simulink model "blank_model_gcm48"  (R2021a)
settings: Solver=FixedStepDiscrete  StartTime=0.0  StopTime=10.0  FixedStep=0.005  RelTol=1e-3  EnableMultiTasking=on
PreLoadFcn:
  | try, model_open; catch, disp('Error occurred while executing model pre-load callback: model_open.m'); disp('Please assure that the MATLAB working directory is set to the model directory before opening.'); end
InitFcn:
  | try, model_open; catch, end
undefined symbols (not defined in the file): dataName, enumName, enumValue, GCM, raptor_get_safe_string, raptor_xcp_function
libraries: Raptor_lib x50, simulink x8
(part 1 of 2)
CloseFcn:
  | try, model_close; catch, end
settings Model: Raptor_Target=GCM-5605B-048-2104  Raptor_Calloc=NonVolatile (EEPROM)  RaptorUIDSize=4  RaptorBuildNum=3  Raptor_ecuaddr=11  Raptor_IsLiteMode=1  Creator=Ben  LastModifiedBy=siddh
settings SolverCC: AlgebraicLoopSolver=TrustRegion
settings DataIOCC: LimitDataPoints=on  SaveFormat=Array  SignalLoggingSaveFormat=ModelDataLogs  ReturnWorkspaceOutputs=off
settings OptimizationCC: DefaultParameterBehavior=Inlined  ExpressionDepthLimit=2147483647  InitFltsAndDblsToZero=on  LifeSpan=1  EfficientTunableParamExpr=on
settings DebuggingCC: SolverPrmCheckMsg=warning  InheritedTsInSrcMsg=none  FcnCallInpInsideContextMsg=warning  StateNameClashWarn=warning  SFUnexpectedBacktrackingDiag=warning  SFNoUnconditionalDefaultTransitionDiag=warning  SFExecutionAtInitializationDiag=none  SFMachineParentedDataDiag=warning  ArithmeticOperatorsInVariantConditions=warning
settings HardwareCC: ProdBitPerPointer=32  ProdBitPerSizeT=32  ProdBitPerPtrDiffT=32  ProdLargestAtomicInteger=Long  ProdLargestAtomicFloat=Double  ProdEndianess=BigEndian  ProdWordSize=32  ProdHWDeviceType=Freescale->MPC55xx  TargetIntDivRoundTo=Zero  TargetEndianess=BigEndian  ProdEqTarget=off
settings ModelReferenceCC: PropagateSignalLabelsOutOfModel=off
settings SFSimCC: SimUseLocalCustomCode=off  MATLABDynamicMemAlloc=off  CustomCodeUndefinedFunction=UseInterfaceOnly
settings RTWCC: Description=Raptor (tm)  SystemTargetFile=raptor.tlc  GenCodeOnly=on  MakeCommand=raptor_make_rtw  TemplateMakefile=raptor.tmf  RTWUseLocalCustomCode=off
settings CodeAppCC: IgnoreCustomStorageClasses=off  MaxIdLength=100  CustomSymbolStrType=$N$R$M  StateflowObjectComments=on  InternalIdentifier=Classic
settings STFCustomTargetCC: GenerateSampleERTMain=on  ModelReferenceCompliant=off  CombineOutputUpdateFcns=on  ERTCustomFileBanners=on  SupportContinuousTime=off  SupportNonInlinedSFcns=off  RemoveResetFunc=on  MATLABClassNameForMDSCustomization=Simulink.SoftwareTarget.ERTCustomization  GRTInterface=off  UseToolchainInfoCompliant=off  SystemTargetFile=raptor.tlc
settings ERTTargetCC: MultiwordLength=2048  GenerateSampleERTMain=on  ModelReferenceCompliant=off  ParMdlRefBuildCompliant=off  CompOptLevelCompliant=off  ConcurrentExecutionCompliant=off  ModelStepFunctionPrototypeControlCompliant=off  CPPClassGenCompliant=off  UseToolchainInfoCompliant=off  ExtModeMexFile=noextcomm  InlinedParameterPlacement=NonHierarchical  ERTCustomFileTemplate=example_file_process.tlc  ConvertIfToSwitch=off  SuppressUnreachableDefaultCases=off
settings ConfigComp: CovMetricSettings=dw  CovSaveCumulativeToWorkspaceVar=on  CovSaveSingleToWorkspaceVar=on  CovExternalEMLEnable=off  CovSFcnEnable=off

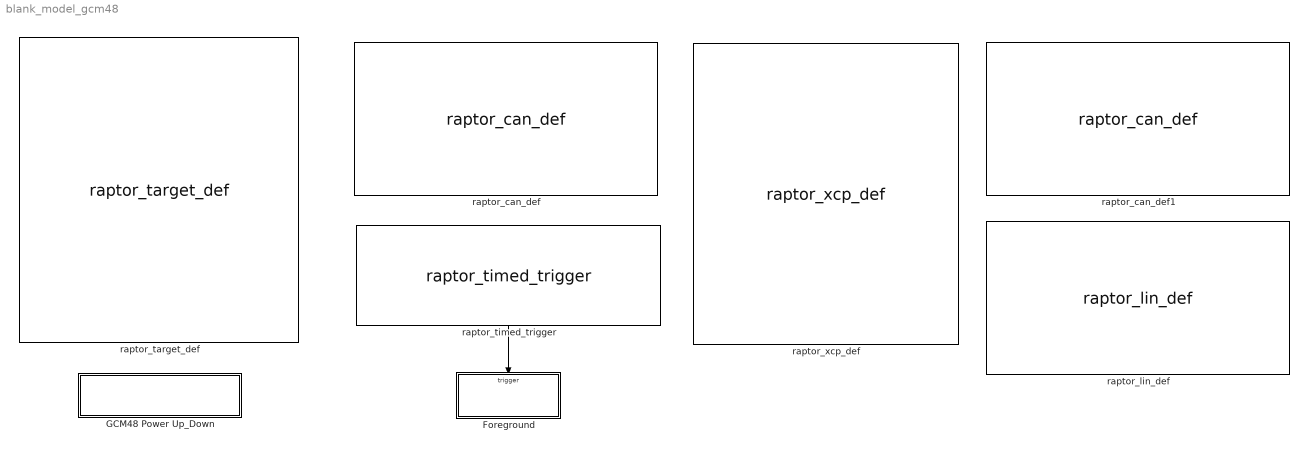
== system blank_model_gcm48 ==
  Foreground : Subsystem  TreatAsAtomicUnit=on
      mask init:
      | handles = get_param(gcb,'PortHandles');
      | portConnectivity = get_param(gcb,'PortConnectivity');
      | for i = 1:length(portConnectivity)
      |     if strcmp(portConnectivity(i).Type,'trigger')
      |         triggerBlk = portConnectivity(i).SrcBlock;
      |         triggerString = get_param(triggerBlk,'trigger');
      |         break;
      |     end
      | end
      | 
      | trigConfBlks = find_system(bdroot,'MaskType','Timed Trigger Configuration Block');
      | trigConfigFound = false;
      | for i = 1:length(trigConfBlks)
      |     if ~isempty(strfind(triggerString,raptor_get_param_eval(trigConfBlks{i},'trigger')))
      |         %if this if statement is met, it means, for example, the text
      |         %"Background" was found in the trigger name of "Backgroundx5"
      |         period_ms = raptor_get_param_eval(trigConfBlks{i},'period');
      |         trigConfigFound = true;
      |         break;
      |     end      
      | end
      | 
      | if ~trigConfigFound %no config defined
      |     switch triggerString
      |         case 'Second'
      |             period_ms = 1000;
      |         case 'Minute'
      |             period_ms = 60*1000;
      |         case 'Foreground'
      |             period_ms = 10;
      |         case 'Background'
      |             period_ms = 100;
      |     end
      | end    
      | 
      | switch triggerString(end-1:end)
      |     case 'x2' %Fgnd or Bgnd slowed by a factor of 2
      |         mult = 2;
      |     case 'x5'
      |         mult = 5;
      |     case '10'
      |         mult = 10;
      |     case '20'
      |         mult = 20;
      |     otherwise
      |         mult = 1;
      | end
      | samptime = period_ms/1000*mult;
      settings: RTWSystemCode=Nonreusable function
      mask Display: disp(['Sample Time:\n' num2str(samptime)])
  GCM48 Power Up_Down : Subsystem  mask{group='Diagnostics | Power Up_Down'}
  raptor_can_def : Raptor_lib/CAN/raptor_can_def  canBus='CAN1'  resourceValues=CAN1|CAN2|CAN3|CAN4|CAN5|CAN6|(None)  resource=CAN1  baudRateValues=33k|50k|100k|125k|200k|250k|333k|500k|667k|800k|1000k  baudRate=500k  enable_baud_rate_config=0  sim_func_name='ConfigureCANBaudRate'  createButton=[]  txQueueSize=20  rxQueueSize=16
      settings: SourceProductName=Raptor
  raptor_can_def1 : Raptor_lib/CAN/raptor_can_def  canBus='CAN2'  resourceValues=CAN1|CAN2|CAN3|CAN4|CAN5|CAN6|(None)  resource=CAN2  baudRateValues=125k|250k|500k|1000k  baudRate=500k  enable_baud_rate_config=0  sim_func_name='ConfigureCANBaudRate'  createButton=[]  txQueueSize=20  rxQueueSize=16
      settings: SourceProductName=Raptor
  raptor_lin_def : Raptor_lib/LIN/raptor_lin_def  linBus='LIN2'  resourceValues=LIN1|LIN2|LIN3|(None)  resource=LIN2  baudRateValues=1200|2400|4800|9600|10000|10400|19200  baudRate=10400  ldfFile='lin_example.ldf'  master=''  chooseLdf=[]
      settings: SourceProductName=Raptor
  raptor_target_def : Raptor_lib/Configuration/raptor_target_def  targetValues=BCM-5646-48-1404|DISP-VC128-1901|DISP-VC320L-1402|DISP-VC320-1204|DISP-VC800-1402|DISP-VC500-1904|DISP-VC700-2003|DISP-VC300R-2004|GCM-5634M-070-1459|GCM-5634M-070-1559|GCM-5634M-070-1562|ECM-1793-196-1503|GCM-1793-196-1503|GCM-5605B-048-1906|GCM-5605B-048-2104|GCM-5607B-80-1901|GCM-5607B-80-1903|GCM-5607B-80-2001|RCM-5743R-080-2005|RCM-5743R-080-2106|UAS-5743R-047-2102|UAS-5743R-047-2107|GCM-5746R-048-1902|RCM-58NN-112-2007|HCM-5604-36-1303|HCM-5604-36-1702  target=GCM-5605B-048-2104  simpack=0  simulator=0  heap=4*1024  stack=2*1024  fgndStack=3*1024  bgndStack=2*1024  idleStack=1024  intStack=1536  sdStack=1024  appStack=1024  ecuaddr=11  uds_server_addr_ext=0  uds_server_addr=hex2dec('600')  uds_client_addr=hex2dec('650')  callocValues=Constant (FLASH)|NonVolatile (EEPROM)  calloc=NonVolatile (EEPROM)  compilerValues=S32 Design Studio for Power Architecture Version 2017.R1  compiler=S32 Design Studio for Power Architecture Version 2017.R1  setFileName=0  exeName=[raptor_get_safe_string(bdroot) '_']  addBuildNum=1  minVerChars=3  extraOutput=0  buildLocationValues=Raptor Default|Model Directory|User Defined  buildLocation=Model Directory  exeLocation=''  a2lLocation=''  rpgLocation=''
      settings: SourceProductName=Raptor
  raptor_timed_trigger : Raptor_lib/Triggers/raptor_timed_trigger  triggerValues=Foreground|Foregroundx2|Foregroundx5|Foregroundx10|Foregroundx20|Background|Backgroundx2|Backgroundx5|Backgroundx10|Backgroundx20|Second|Minute  trigger=Foreground  inherited=0  alwaysEnabled=1  triggerPriority=0  triggerName=ooqlV
      settings: SourceProductName=Raptor
  raptor_xcp_def : Raptor_lib/Configuration/raptor_xcp_def  canBus='CAN1'  bcID=hex2dec('100')  bcID_TypeValues=Standard|Extended  bcID_Type=Standard  rxID=hex2dec('200')  rxID_TypeValues=Standard|Extended  rxID_Type=Standard  txID=hex2dec('300')  txID_TypeValues=Standard|Extended  txID_Type=Standard  daqRates=[10 50 100 500 1000]  numODTs=20  genCANAPE=0  genVISION=0  securityValues=Standard|None|Custom User Defined  security=Standard  dllName=raptor_XCPSecurity.dll  accessValues=4|3|2|1  access=1  bcStorageValues=[]  bcStorage=Calibration  txStorageValues=[]  txStorage=Calibration  rxStorageValues=[]  rxStorage=Calibration
      settings: SourceProductName=Raptor
  wires:
  raptor_timed_trigger/1 -> Foreground/Trigger

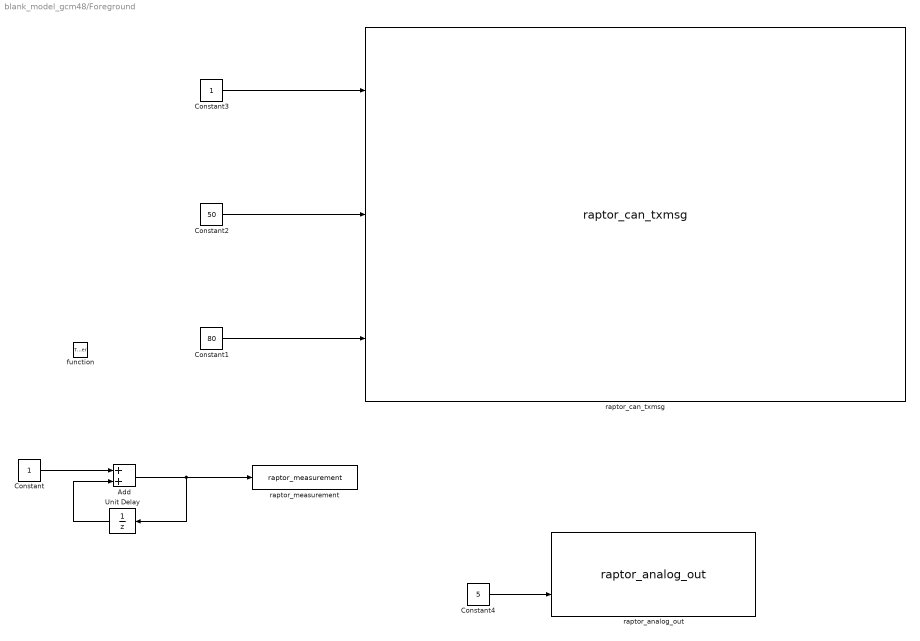
== system blank_model_gcm48/Foreground ==
  function : TriggerPort  TriggerType=function-call  VariantControl=Variant
  Add : Sum
  Constant : Constant
  Constant1 : Constant  Value=80
  Constant2 : Constant  Value=50
  Constant3 : Constant
  Constant4 : Constant  Value=5
  Unit Delay : UnitDelay  SampleTime=-1  HasFrameUpgradeWarning=on
  raptor_analog_out : Raptor_lib/Input & Output/raptor_analog_out  resourceValues=[]  resource=[]
      settings: SourceProductName=Raptor
  raptor_can_txmsg : Raptor_lib/CAN/raptor_can_txmsg  canDefinition=struct('dbcFile', 'can_example.dbc','message', 'ExampleMsgTxExtended','comment', 'Example message','signals', {{'Enable','EngineSpeed','EngineTemperature'}},'enabled', [ 1 1 1;],'scaled', [ 1 1 1;],'canBus', '''CAN1''','messageID', [ 777;],'idMask', [ 536870911;],'payloadMask', [],'payloadValue', [],'period', [ 0;],'mailbox', '','queueSize', [ 1;],'label', [ 0;],'ver', [ 2;],'showID', [ 0;],'showRaw', [ 0;],'showRawMsg', [ 0;],'fill', [ 0;],'editID', [ 0;],'signalOrder', [ 1;],'signalAscDes', [ 1;])  canBus='CAN1'  queueSize=1  payloadMask=[]  payloadValue=[]  period=0  showID=0  label=0  idMask=hex2dec('1FFFFFFF')  fill=0  id=777  showRaw=0  signalOrder=1  signalInfo={{struct('Name', 'Enable','Startbit', [ 0;],'SignalSize', [ 1;],'ByteOrder', 'BigEndian','ValueType', 'UNSIGNED','Class', 'uint8','Signed', [ 0;],'Factor', [ 1;],'Offset', [ 0;],'Min', [ 0;],'Max', [ 1;],'Units', '','Comment', '','StartBit', [ 0;]),struct('Name', 'EngineSpeed','Startbit', [ 0;],'SignalSize', [ 16;],'ByteOrder', 'BigEndian','ValueType', 'UNSIGNED','Class', 'uint16','Signed', [ 0;],'Factor', [ 0.1;],'Offset', [ 0;],'Min', [ 0;],'Max', [ 6500;],'Units', 'rpm','Comment', '','StartBit', [ 16;]),struct('Name', 'EngineTemperature','Startbit', [ 0;],'SignalSize', [ 16;],'ByteOrder', 'BigEndian','ValueType', 'UNSIGNED','Class', 'uint16','Signed', [ 0;],'Factor', [ 0.01;],'Offset', [ -40;],'Min', [ -40;],'Max', [ 500;],'Units', 'degC','Comment', '','StartBit', [ 32;])}}
      settings: SourceProductName=Raptor
  raptor_measurement : Raptor_lib/Data Storage/raptor_measurement  paramName='Counter'  nameSource=Parameter  calDispType=Number  calEnum={'False', 'True'}  calGain=1.0  calOffset=0.0  calMax=inf  calMin=-inf  calFormat='-1'  calUnit=''  calHelp=''  calAccess=4  calFunction=raptor_xcp_function(gcb)  calVisible=on
      settings: SourceProductName=Raptor
  wires:
  Constant/1 -> Add/1
  Add/1 -> raptor_measurement/1, Unit Delay/1
  Unit Delay/1 -> Add/2
  Constant1/1 -> raptor_can_txmsg/3
  Constant2/1 -> raptor_can_txmsg/2
  Constant3/1 -> raptor_can_txmsg/1
  Constant4/1 -> raptor_analog_out/2

== system blank_model_gcm48/GCM48 Power Up_Down ==
  Background : Subsystem  mask{group='System | Power Up_Down'}
      mask init: same as blank_model_gcm48/Foreground
      mask Display: disp(['Sample Time:\n' num2str(samptime)])
  raptor_timed_trigger : Raptor_lib/Triggers/raptor_timed_trigger  triggerValues=Foreground|Foregroundx2|Foregroundx5|Foregroundx10|Foregroundx20|Background|Backgroundx2|Backgroundx5|Backgroundx10|Backgroundx20|Second|Minute  trigger=Background  inherited=0  alwaysEnabled=1  triggerPriority=50  triggerName=BGND_9AY_V
      settings: SourceProductName=Raptor
  wires:
  raptor_timed_trigger/1 -> Background/Trigger

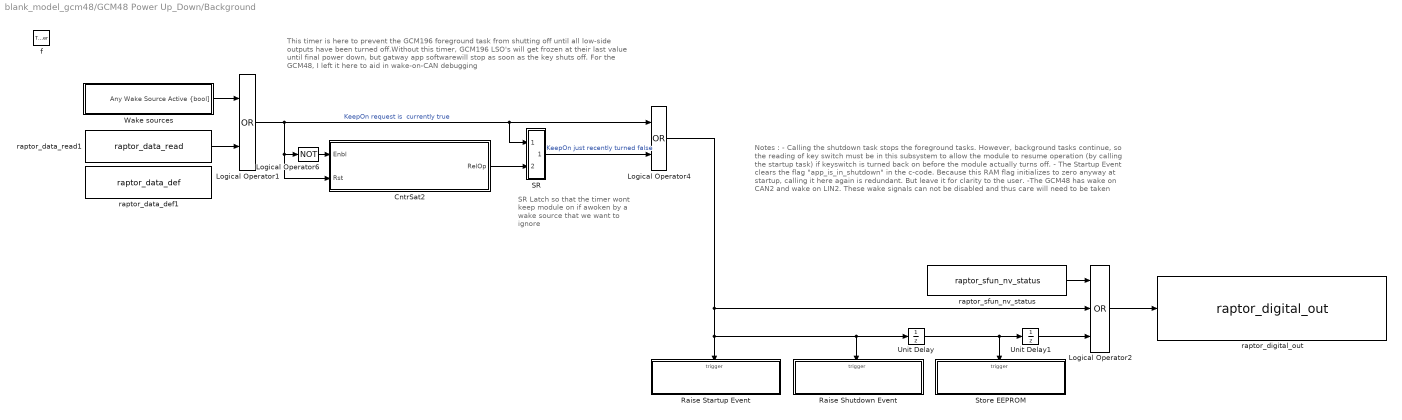
== system blank_model_gcm48/GCM48 Power Up_Down/Background ==
  note: SR Latch so that the timer wont keep module on if awoken by a wake source that we want to ignore
  note: Notes :
      | - Calling the shutdown task stops the foreground tasks. However, background tasks continue, so the reading of key switch must be in this subsystem to allow the module
      | to resume operation (by calling the startup task) if keyswitch is turned back on before the module actually turns off.
      | - The Startup Event clears the flag "app_is_in_shutdown" in the c-code. Because this RAM flag initializes to zero anyway at startup, calling it here again is redundant. But leave it for clarity to the user.
      |
      | -The GCM48 has wake on CAN2 and wake on LIN2. These wake signals can not be disabled and thus care will need to be taken
  note: This timer is here to prevent the GCM196 foreground task from shutting off until all low-side outputs have been turned off.Without this timer, GCM196 LSO's will get frozen at their last value until final power down, but gatway app softwarewill stop as soon as the key shuts off.
      |
      | For the GCM48, I left it here to aid in wake-on-CAN debugging
  f : TriggerPort  TriggerType=function-call  VariantControl=Variant  ZeroCross=off
  CntrSat2 : Subsystem  mask(CntrSat){init=0, inc=1, typ=uint32, relop=>=, th_nam='Wake_DlyStopOfFgndTaskTime', th_help='When key switch goes false, the foreground task will be held on for this amount of time to allow low side outputs to turn off', th_units='sec', th_gain=samptime, th_group=group}
      mask prompts: init "Initial Value (after a reset)"; inc "Increment"; typ "Data Type"; relop "Relational Operator"; th_nam "Thresh. Name"; th_help "Thresh. Help Text"; th_units "Thresh. Units"; th_gain "Thresh. Gain"; th_group "Thresh. Group"
      mask init:
      | cb = gcb;
      | 
      | % --- Parameter Setting
      | set_param([cb '/Relational Operator'], 'Operator', relop);
      | set_param([cb '/raptor_adjustment'], 'dataType', typ);
      | set_param([cb '/Constant'], 'OutDataTypeStr', typ);
      | set_param([cb '/Constant1'], 'OutDataTypeStr', typ);
      | 
      | % --- Precision
      | try
      |     th_gain_eval = raptor_get_param_eval(th_gain);
      |     inc_eval = raptor_get_param_eval(inc);
      |     prec = SamptimePrec(th_gain_eval * inc_eval);
      | catch
      |     prec = '';
      | end
      mask TypeOptions typ: double | single | int8 | uint8 | int16 | uint16 | int32 | uint32 | boolean
      mask TypeOptions relop: == | >= | >
      mask Display: disp(['Counter\n' typ '\n' relop ' ' th_nam]);
  Logical Operator1 : Logic  Operator=OR  OutDataTypeStr=boolean
  Logical Operator2 : Logic  Operator=OR  Inputs=3  OutDataTypeStr=boolean
  Logical Operator4 : Logic  Operator=OR  OutDataTypeStr=boolean
  Logical Operator6 : Logic  Operator=NOT  OutDataTypeStr=boolean
  Raise Shutdown Event : Subsystem  TreatAsAtomicUnit=on
  Raise Startup Event : Subsystem  TreatAsAtomicUnit=on
  SR : Subsystem  mask(SetRst){init=0}
      mask prompts: init "Initial Condition (of output):"
      mask Display:
      | port_label('input', 1, 'S');
      | port_label('input', 2, 'R');
  Store EEPROM : Subsystem  TreatAsAtomicUnit=on
  Unit Delay : UnitDelay  SampleTime=-1  HasFrameUpgradeWarning=on
  Unit Delay1 : UnitDelay  SampleTime=-1  HasFrameUpgradeWarning=on
  Wake sources : Subsystem
  raptor_data_def1 : Raptor_lib/Data Storage/raptor_data_def  dataName='KeepModuleOn'  initValue=0  dataType=boolean  storage=Volatile (RAM)  calVisible=on  calType=Measurement  calDispType=Number  calEnum={'False', 'True'}  calGain=1.0  calOffset=0  calMin=-Inf  calMax=Inf  calFormat='-1'  calUnit='Bool'  calHelp='Boolean indicating module to be kept on'  calAccess=2  calFunction=group  calDispHeaders=off  calColHeaders={'Col1' 'Col2' 'Col3'}  calRowHeaders={'Row1' 'Row2' 'Row3'}
      settings: SourceProductName=Raptor
  raptor_data_read1 : Raptor_lib/Data Storage/raptor_data_read  dataName='KeepModuleOn'  dataShape=Scalar  idxSource=Input  idxRow=1  idxCol=1
      settings: SourceProductName=Raptor
  raptor_digital_out : Raptor_lib/Input & Output/raptor_digital_out  resourceValues=OUTPUT9|OUTPUT21|OUTPUT22|OUTPUT23|OUTPUT24|(None)|OUTPUT1|OUTPUT2|OUTPUT3|OUTPUT4|OUTPUT5|OUTPUT6|OUTPUT7|OUTPUT8|OUTPUT10|OUTPUT11|OUTPUT25|OUTPUT26|OUTPUT27|OUTPUT28|OUTPUT29|OUTPUT30|OUTPUT31|OUTPUT32|OUTPUT33|OUTPUT34|OUTPUT35|OUTPUT36|OUTPUT37|OUTPUT38|OUTPUT39|OUTPUT40|OUTPUT41|OUTPUT42|OUTPUT43|OUTPUT44|OUTPUT45|OUTPUT46|OUTPUT47|OUTPUT48|POWER_HOLD  resource=POWER_HOLD  driverTypeValues=(None)  driverType=(None)
      settings: SourceProductName=Raptor
  raptor_sfun_nv_status : Raptor_lib/Data Storage/raptor_sfun_nv_status  showStatus=Store In Progess
      settings: SourceProductName=Raptor
  wires:
  Wake sources/1("Any Wake Source Active {bool]") -> Logical Operator1/1
  SR/1(Bool) -> Logical Operator4/2  "KeepOn just recently turned false"
  Logical Operator6/1 -> CntrSat2/1(Enbl)
  Logical Operator1/1 -> CntrSat2/2(Rst), Logical Operator6/1, SR/1(Set), Logical Operator4/1  "KeepOn request is  currently true"
  CntrSat2/1(RelOp) -> SR/2(Rst)
  Logical Operator4/1 -> Logical Operator2/2, Raise Startup Event/Trigger, Unit Delay/1, Raise Shutdown Event/Trigger
  Unit Delay/1 -> Unit Delay1/1, Store EEPROM/Trigger
  raptor_sfun_nv_status/1 -> Logical Operator2/1
  Logical Operator2/1 -> raptor_digital_out/1
  Unit Delay1/1 -> Logical Operator2/3
  raptor_data_read1/1 -> Logical Operator1/2

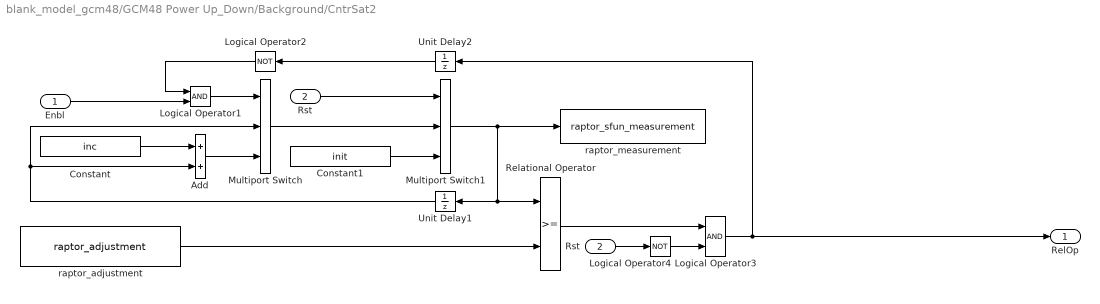
== system blank_model_gcm48/GCM48 Power Up_Down/Background/CntrSat2 ==
  Enbl : Inport
  Rst : Inport  Port=2
  Add : Sum  InputSameDT=on  OutDataTypeStr=Inherit: Same as first input
  Constant : Constant  Value=inc  OutDataTypeStr=uint32
  Constant1 : Constant  Value=init  OutDataTypeStr=uint32
  Logical Operator1 : Logic  OutDataTypeStr=boolean
  Logical Operator2 : Logic  Operator=NOT  Inputs=1  OutDataTypeStr=boolean
  Logical Operator3 : Logic  OutDataTypeStr=boolean
  Logical Operator4 : Logic  Operator=NOT  Inputs=1  OutDataTypeStr=boolean
  Multiport Switch : MultiPortSwitch  DataPortOrder=Zero-based contiguous  Inputs=2  zeroidx=on  InputSameDT=on
  Multiport Switch1 : MultiPortSwitch  DataPortOrder=Zero-based contiguous  Inputs=2  zeroidx=on  InputSameDT=on
  Relational Operator : RelationalOperator  OutDataTypeStr=boolean  RndMeth=Nearest
  "Rst " : InportShadow  Port=2
  Unit Delay1 : UnitDelay  InitialCondition=init  SampleTime=-1  HasFrameUpgradeWarning=on
  Unit Delay2 : UnitDelay  InitialCondition=boolean(0)  SampleTime=-1  HasFrameUpgradeWarning=on
  raptor_adjustment : Raptor_lib/Data Storage/raptor_adjustment  paramName=th_nam  nameSource=Parameter  initValue=.1 / th_gain  dataType=uint32  storage=Calibration  calDispType=Number  calEnum={'Disabled', 'Enabled'}  calGain=th_gain  calOffset=0  calMax=inf  calMin=-inf  calFormat='0.3'  calUnit=th_units  calHelp=th_help  calAccess=4  calFunction=th_group  calDispHeaders=off  calColHeaders={'Col1' 'Col2' 'Col3'}  calRowHeaders={'Row1' 'Row2' 'Row3'}
      settings: SourceProductName=Raptor
  raptor_measurement : S-Function  FunctionName=raptor_sfun_measurement  Parameters=char({dataName,''}), uint8(calDispType), char(enumName), int32(enumValue), double(calGain), double(calOffset), double(calMax), double(calMin), char(calUnit), char(calHelp), char(calFormat), char(calFunction), char(calAccess)  SFunctionDeploymentMode=off  EnableBusSupport=off  mask(Measurement){paramName=[th_nam(1:end-3) 'Tmr'], nameSource=Parameter, calDispType=Number, calEnum={'False', 'True'}, calGain=th_gain, calOffset=0.0, calMax=inf, calMin=-inf, calFormat='0.3', calUnit=th_units, calHelp=['time that gets compared to ' th_nam], calAccess=4, calFunction=th_group, calVisible=on}
      mask prompts: paramName "Name"; nameSource "Name Source"; calDispType "Display as"; calEnum "Enumeration Definition"; calGain "Gain"; calOffset "Offset"; calMax "Max"; calMin "Min"; calFormat "Display Decimal Places"; calUnit "Unit Text"; calHelp "Help Text"; calAccess "Access Level"; calFunction "Function"; calVisible "Visible in Cal"
      mask help: This block is used to display a value in the calibration tool.
      mask init:
      | raptor_sfun_measurement_maskInit;
      settings: MoveFcn=raptor_icon_redraw(gcb);
      mask Help: eval('raptor_help(''raptor_measurement'');')
      mask TypeOptions nameSource: Parameter | Input Wire
      mask Callback nameSource: raptor_sfun_measurement_dlgCb(gcb, 'nameSource');
      mask TypeOptions calDispType: Number | Enumeration | String
      mask Callback calDispType: raptor_sfun_measurement_dlgCb(gcb, 'calDispType');
      mask TypeOptions calAccess: 4 | 3 | 2 | 1
      mask Display: raptor_sfun_measurement_icon;
  RelOp : Outport  VectorParamsAs1DForOutWhenUnconnected=off
  wires:
  "Rst "/1 -> Logical Operator4/1
  Logical Operator4/1 -> Logical Operator3/2
  Relational Operator/1 -> Logical Operator3/1
  Multiport Switch1/1 -> Relational Operator/1, Unit Delay1/1, raptor_measurement/1
  Logical Operator2/1 -> Logical Operator1/1
  Constant1/1 -> Multiport Switch1/3
  Multiport Switch/1 -> Multiport Switch1/2
  Constant/1 -> Add/1
  Unit Delay1/1 -> Multiport Switch/2, Add/2
  Add/1 -> Multiport Switch/3
  Logical Operator1/1 -> Multiport Switch/1
  Enbl/1 -> Logical Operator1/2
  raptor_adjustment/1 -> Relational Operator/2
  Logical Operator3/1 -> RelOp/1, Unit Delay2/1
  Rst/1 -> Multiport Switch1/1
  Unit Delay2/1 -> Logical Operator2/1

== system blank_model_gcm48/GCM48 Power Up_Down/Background/Raise Shutdown Event ==
  init state = 1 to trigger at wakeup if awoken by a wake source that we want to ignore : TriggerPort  TriggerType=falling  VariantControl=Variant  InitialTriggerSignalState=positive
  Constant : Constant  Value=boolean(1)
  Function-Call Generator : simulink/Ports & Subsystems/Function-Call Generator  sample_time=-1  numberOfIterations=1  DisallowWideOutput=off
  raptor_data_def : Raptor_lib/Data Storage/raptor_data_def  dataName='FgndTasksStopped'  initValue=0  dataType=boolean  storage=Volatile (RAM)  calVisible=on  calType=Measurement  calDispType=Number  calEnum={'False', 'True'}  calGain=1.0  calOffset=0  calMin=-Inf  calMax=Inf  calFormat='-1'  calUnit='Bool'  calHelp='Boolean indicating foreground tasks stopped'  calAccess=4  calFunction=group  calDispHeaders=off  calColHeaders={'Col1' 'Col2' 'Col3'}  calRowHeaders={'Row1' 'Row2' 'Row3'}
      settings: SourceProductName=Raptor
  raptor_data_write : Raptor_lib/Data Storage/raptor_data_write  dataName='FgndTasksStopped'  dataShape=Scalar  idxSource=Input Port  idxRow=1  idxCol=1
      settings: SourceProductName=Raptor
  raptor_shutdown : Raptor_lib/Triggers/raptor_shutdown  null=0
      settings: SourceProductName=Raptor
  wires:
  Function-Call Generator/1 -> raptor_shutdown/Trigger
  Constant/1 -> raptor_data_write/1

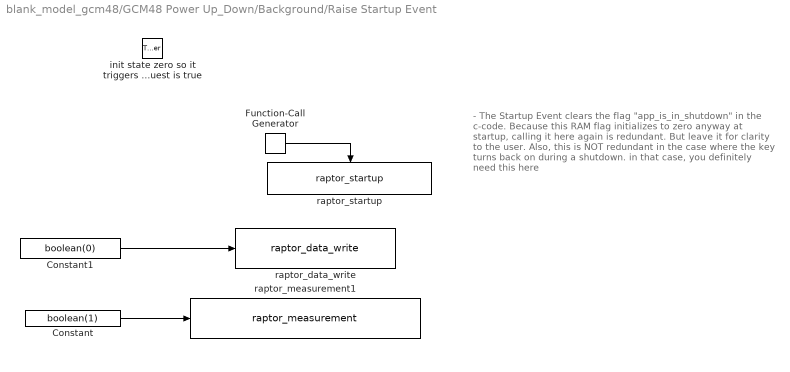
== system blank_model_gcm48/GCM48 Power Up_Down/Background/Raise Startup Event ==
  note: - The Startup Event clears the flag "app_is_in_shutdown" in the c-code. Because this RAM flag initializes to zero anyway at startup, calling it here again is redundant. But leave it for clarity to the user.
      |
      | Also, this is NOT redundant in the case where the key turns back on during a shutdown. in that case, you definitely need this here
  init state zero so it triggers at wake if wake request is true : TriggerPort  VariantControl=Variant  InitialTriggerSignalState=zero  PortDimensions=1
  Constant : Constant  Value=boolean(1)
  Constant1 : Constant  Value=boolean(0)
  Function-Call Generator : simulink/Ports & Subsystems/Function-Call Generator  sample_time=-1  numberOfIterations=1  DisallowWideOutput=off
  raptor_data_write : Raptor_lib/Data Storage/raptor_data_write  dataName='FgndTasksStopped'  dataShape=Scalar  idxSource=Input Port  idxRow=1  idxCol=1
      settings: SourceProductName=Raptor
  raptor_measurement1 : Raptor_lib/Data Storage/raptor_measurement  paramName='Wake_Debug_StartupEventRaised'  nameSource=Parameter  calDispType=Number  calEnum={'False', 'True'}  calGain=1.0  calOffset=0.0  calMax=inf  calMin=-inf  calFormat='-1'  calUnit=''  calHelp=''  calAccess=4  calFunction=group  calVisible=on
      settings: SourceProductName=Raptor
  raptor_startup : Raptor_lib/Triggers/raptor_startup  null=0
      settings: SourceProductName=Raptor
  wires:
  Constant1/1 -> raptor_data_write/1
  Constant/1 -> raptor_measurement1/1
  Function-Call Generator/1 -> raptor_startup/Trigger

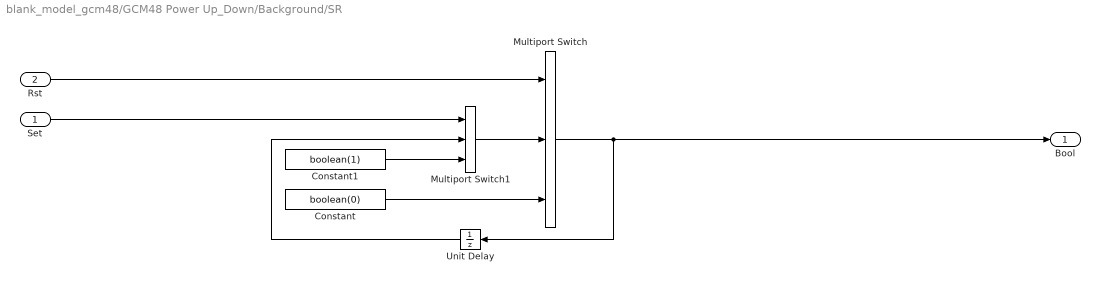
== system blank_model_gcm48/GCM48 Power Up_Down/Background/SR ==
  Set : Inport
  Rst : Inport  Port=2
  Constant : Constant  Value=boolean(0)
  Constant1 : Constant  Value=boolean(1)
  Multiport Switch : MultiPortSwitch  DataPortOrder=Zero-based contiguous  Inputs=2  zeroidx=on
  Multiport Switch1 : MultiPortSwitch  DataPortOrder=Zero-based contiguous  Inputs=2  zeroidx=on
  Unit Delay : UnitDelay  InitialCondition=init  SampleTime=-1  HasFrameUpgradeWarning=on
  Bool : Outport  VectorParamsAs1DForOutWhenUnconnected=off
  wires:
  Multiport Switch1/1 -> Multiport Switch/2
  Constant1/1 -> Multiport Switch1/3
  Constant/1 -> Multiport Switch/3
  Rst/1 -> Multiport Switch/1
  Set/1 -> Multiport Switch1/1
  Multiport Switch/1 -> Bool/1, Unit Delay/1
  Unit Delay/1 -> Multiport Switch1/2

== system blank_model_gcm48/GCM48 Power Up_Down/Background/Store EEPROM ==
  Trigger : TriggerPort  TriggerType=falling  VariantControl=Variant
  Function-Call Generator : simulink/Ports & Subsystems/Function-Call Generator  sample_time=-1  numberOfIterations=1  DisallowWideOutput=off
  raptor_store_nv : Raptor_lib/Data Storage/raptor_store_nv  null=0
      settings: SourceProductName=Raptor
  wires:
  Function-Call Generator/1 -> raptor_store_nv/Trigger

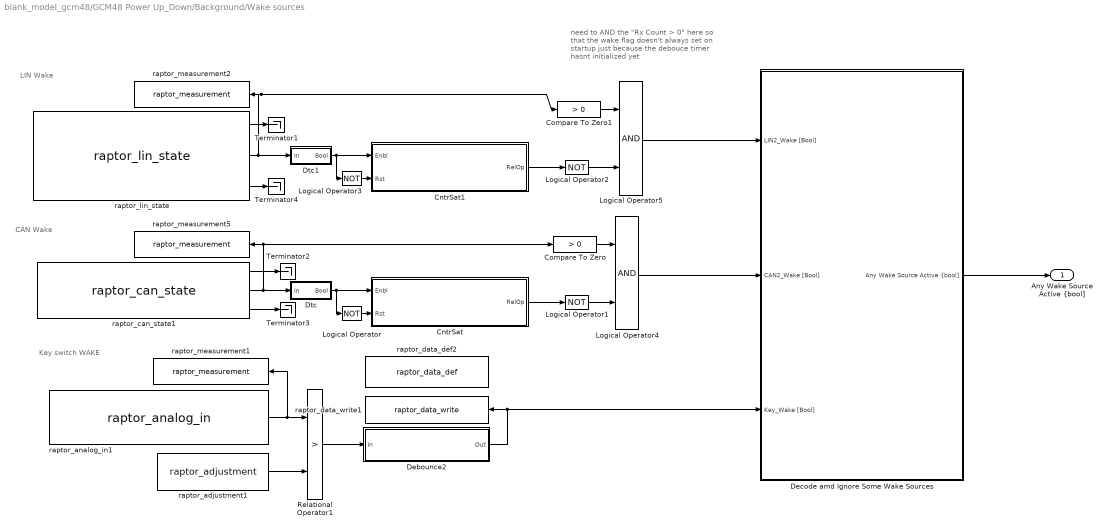
== system blank_model_gcm48/GCM48 Power Up_Down/Background/Wake sources ==
  note: CAN Wake
  note: Key switch WAKE
  note: LIN Wake
  note: need to AND the "Rx Count > 0" here so that the wake flag doesn't always set on startup just because the debouce timer hasnt initialized yet
  CntrSat : Subsystem  mask(CntrSat){init=0, inc=1, typ=uint32, relop=>=, th_nam='Wake_CAN2_SleepDelayTime', th_help='make sure this is long enough that we dont trigger a ton of EEPROM writes between messages', th_units='sec', th_gain=samptime, th_group=group}
      mask prompts: init "Initial Value (after a reset)"; inc "Increment"; typ "Data Type"; relop "Relational Operator"; th_nam "Thresh. Name"; th_help "Thresh. Help Text"; th_units "Thresh. Units"; th_gain "Thresh. Gain"; th_group "Thresh. Group"
      mask init: same as blank_model_gcm48/GCM48 Power Up_Down/Background/CntrSat2
      mask TypeOptions typ: double | single | int8 | uint8 | int16 | uint16 | int32 | uint32 | boolean
      mask TypeOptions relop: == | >= | >
      mask Display: disp(['Counter\n' typ '\n' relop ' ' th_nam]);
  CntrSat1 : Subsystem  mask(CntrSat){init=0, inc=1, typ=uint32, relop=>=, th_nam='Wake_LIN2_SleepDelayTime', th_help='make sure this is long enough that we dont trigger a ton of EEPROM writes between messages', th_units='sec', th_gain=samptime, th_group=group}
      mask prompts: init "Initial Value (after a reset)"; inc "Increment"; typ "Data Type"; relop "Relational Operator"; th_nam "Thresh. Name"; th_help "Thresh. Help Text"; th_units "Thresh. Units"; th_gain "Thresh. Gain"; th_group "Thresh. Group"
      mask init: same as blank_model_gcm48/GCM48 Power Up_Down/Background/CntrSat2
      mask TypeOptions typ: double | single | int8 | uint8 | int16 | uint16 | int32 | uint32 | boolean
      mask TypeOptions relop: == | >= | >
      mask Display: disp(['Counter\n' typ '\n' relop ' ' th_nam]);
  Compare To Zero : simulink/Logic and Bit Operations/Compare To Zero  relop=>  OutDataTypeStr=boolean
  Compare To Zero1 : simulink/Logic and Bit Operations/Compare To Zero  relop=>  OutDataTypeStr=boolean
  Debounce2 : Subsystem
  Decode amd Ignore Some Wake Sources : Subsystem
  Dtc : Subsystem  mask(Dtc){init=0, relop===}
      mask prompts: init "Initial Condition (of input):"; relop "Relational Operator"
      mask init:
      | cb = gcb;
      | 
      | % --- Parameter Setting
      | set_param([cb '/Relational Operator'], 'Operator', relop);
      mask TypeOptions relop: == | ~= | < | <= | >= | >
      mask Display: disp(['U ' relop ' U/z']);
  Dtc1 : Subsystem  mask(Dtc){init=0, relop===}
      mask prompts: init "Initial Condition (of input):"; relop "Relational Operator"
      mask init:
      | cb = gcb;
      | 
      | % --- Parameter Setting
      | set_param([cb '/Relational Operator'], 'Operator', relop);
      mask TypeOptions relop: == | ~= | < | <= | >= | >
      mask Display: disp(['U ' relop ' U/z']);
  Logical Operator{,1..3} (4 alike) : Logic  Operator=NOT  AllPortsSameDT=off  OutDataTypeStr=boolean
  Logical Operator4 : Logic  AllPortsSameDT=off  OutDataTypeStr=boolean
  Logical Operator5 : Logic  AllPortsSameDT=off  OutDataTypeStr=boolean
  Relational Operator1 : RelationalOperator  Operator=>  OutDataTypeStr=boolean  RndMeth=Simplest
  Terminator{1..4} (4 alike) : Terminator
  raptor_adjustment1 : Raptor_lib/Data Storage/raptor_adjustment  paramName='WAKE_INPUT1_Threshold'  nameSource=Parameter  initValue=1200  dataType=uint16  storage=NonVolatile (EEPROM)  calDispType=Number  calEnum={'False', 'True'}  calGain=1  calOffset=0.0  calMax=inf  calMin=-inf  calFormat='-1'  calUnit='V'  calHelp='The value of WAKE_INPUT1 analog to set key switch to true.'  calAccess=4  calFunction=group  calDispHeaders=off  calColHeaders={'Col1' 'Col2' 'Col3'}  calRowHeaders={'Row1' 'Row2' 'Row3'}
      settings: SourceProductName=Raptor
  raptor_analog_in1 : Raptor_lib/Input & Output/raptor_analog_in  resourceValues=DG1|DG2|DG3|DG4|AN1|AN2|AN3|AN4|AN5|AN6|AN7|AN8|AN9|AN10|AN11|AN12|WAKE_INPUT1|(None)  resource=WAKE_INPUT1  pullUDValues=[]  pullUD=[]  rangeValues=[]  range=[]  filterrateValues=[]  filterrate='RAPTOR MASK DEFAULT'  resolutionValues=[]  resolution=[]
      settings: SourceProductName=Raptor
  raptor_can_state1 : Raptor_lib/CAN/raptor_can_state  resourceValues=CAN1|CAN2|CAN3|CAN4|CAN5|CAN6|(None)  resource=CAN2  errOut='RAPTOR MASK DEFAULT'
      settings: SourceProductName=Raptor
  raptor_data_def2 : Raptor_lib/Data Storage/raptor_data_def  dataName='KeySw_Bgnd'  initValue=0  dataType=boolean  storage=Volatile (RAM)  calVisible=on  calType=Measurement  calDispType=Number  calEnum={'False', 'True'}  calGain=1.0  calOffset=0  calMin=-Inf  calMax=Inf  calFormat='-1'  calUnit='Bool'  calHelp='Key switch reading from background task'  calAccess=4  calFunction=group  calDispHeaders=off  calColHeaders={'Col1' 'Col2' 'Col3'}  calRowHeaders={'Row1' 'Row2' 'Row3'}
      settings: SourceProductName=Raptor
  raptor_data_write1 : Raptor_lib/Data Storage/raptor_data_write  dataName='KeySw_Bgnd'  dataShape=Scalar  idxSource=Input Port  idxRow=1  idxCol=1
      settings: SourceProductName=Raptor
  raptor_lin_state : Raptor_lib/LIN/raptor_lin_state  linBus='LIN2'
      settings: SourceProductName=Raptor
  raptor_measurement1 : Raptor_lib/Data Storage/raptor_measurement  paramName='Wake_INPUT1_Vlts'  nameSource=Parameter  calDispType=Number  calEnum={'False', 'True'}  calGain=38/4096  calOffset=0.0  calMax=inf  calMin=-inf  calFormat='-1'  calUnit=''  calHelp=''  calAccess=4  calFunction=group  calVisible=on
      settings: SourceProductName=Raptor
  raptor_measurement2 : Raptor_lib/Data Storage/raptor_measurement  paramName='Wake_LIN2_RxCount'  nameSource=Parameter  calDispType=Number  calEnum={'False', 'True'}  calGain=1.0  calOffset=0.0  calMax=inf  calMin=-inf  calFormat='-1'  calUnit=''  calHelp=''  calAccess=4  calFunction=group  calVisible=on
      settings: SourceProductName=Raptor
  raptor_measurement5 : Raptor_lib/Data Storage/raptor_measurement  paramName='Wake_CAN2_RxCount'  nameSource=Parameter  calDispType=Number  calEnum={'False', 'True'}  calGain=1.0  calOffset=0.0  calMax=inf  calMin=-inf  calFormat='-1'  calUnit=''  calHelp=''  calAccess=4  calFunction=group  calVisible=on
      settings: SourceProductName=Raptor
  "Any Wake Source Active {bool]" : Outport  VectorParamsAs1DForOutWhenUnconnected=off
  wires:
  Logical Operator5/1 -> Decode amd Ignore Some Wake Sources/1(LIN2_Wake [Bool])
  Logical Operator2/1 -> Logical Operator5/2
  Compare To Zero1/1 -> Logical Operator5/1
  Logical Operator4/1 -> Decode amd Ignore Some Wake Sources/2(CAN2_Wake [Bool])
  Compare To Zero/1 -> Logical Operator4/1
  Logical Operator1/1 -> Logical Operator4/2
  Decode amd Ignore Some Wake Sources/1("Any Wake Source Active {bool]") -> "Any Wake Source Active {bool]"/1
  raptor_can_state1/3 -> Terminator3/1
  raptor_adjustment1/1 -> Relational Operator1/2
  raptor_can_state1/1 -> Terminator2/1
  raptor_lin_state/3 -> Terminator4/1
  raptor_lin_state/1 -> Terminator1/1
  CntrSat1/1(RelOp) -> Logical Operator2/1
  Logical Operator/1 -> CntrSat/2(Rst)
  raptor_lin_state/2 -> Dtc1/1(In), raptor_measurement2/1, Compare To Zero1/1
  Logical Operator3/1 -> CntrSat1/2(Rst)
  Dtc1/1(Bool) -> Logical Operator3/1, CntrSat1/1(Enbl)
  Relational Operator1/1 -> Debounce2/1(In)
  Dtc/1(Bool) -> CntrSat/1(Enbl), Logical Operator/1
  CntrSat/1(RelOp) -> Logical Operator1/1
  raptor_analog_in1/1 -> Relational Operator1/1, raptor_measurement1/1
  Debounce2/1(Out) -> raptor_data_write1/1, Decode amd Ignore Some Wake Sources/3(Key_Wake [Bool])
  raptor_can_state1/2 -> raptor_measurement5/1, Compare To Zero/1, Dtc/1(In)

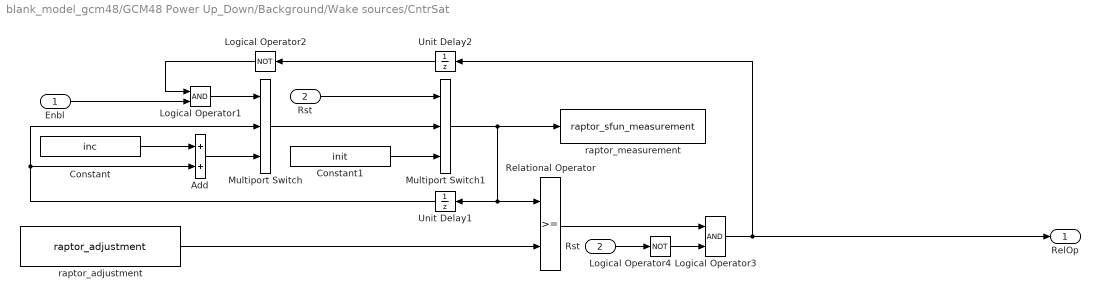
== system blank_model_gcm48/GCM48 Power Up_Down/Background/Wake sources/CntrSat ==
  Enbl : Inport
  Rst : Inport  Port=2
  Add : Sum  InputSameDT=on  OutDataTypeStr=Inherit: Same as first input
  Constant : Constant  Value=inc  OutDataTypeStr=uint32
  Constant1 : Constant  Value=init  OutDataTypeStr=uint32
  Logical Operator1 : Logic  OutDataTypeStr=boolean
  Logical Operator2 : Logic  Operator=NOT  Inputs=1  OutDataTypeStr=boolean
  Logical Operator3 : Logic  OutDataTypeStr=boolean
  Logical Operator4 : Logic  Operator=NOT  Inputs=1  OutDataTypeStr=boolean
  Multiport Switch : MultiPortSwitch  DataPortOrder=Zero-based contiguous  Inputs=2  zeroidx=on  InputSameDT=on
  Multiport Switch1 : MultiPortSwitch  DataPortOrder=Zero-based contiguous  Inputs=2  zeroidx=on  InputSameDT=on
  Relational Operator : RelationalOperator  OutDataTypeStr=boolean  RndMeth=Nearest
  "Rst " : InportShadow  Port=2
  Unit Delay1 : UnitDelay  InitialCondition=init  SampleTime=-1  HasFrameUpgradeWarning=on
  Unit Delay2 : UnitDelay  InitialCondition=boolean(0)  SampleTime=-1  HasFrameUpgradeWarning=on
  raptor_adjustment : Raptor_lib/Data Storage/raptor_adjustment  paramName=th_nam  nameSource=Parameter  initValue=5 / th_gain  dataType=uint32  storage=Calibration  calDispType=Number  calEnum={'Disabled', 'Enabled'}  calGain=th_gain  calOffset=0  calMax=inf  calMin=-inf  calFormat='0.3'  calUnit=th_units  calHelp=th_help  calAccess=4  calFunction=th_group  calDispHeaders=off  calColHeaders={'Col1' 'Col2' 'Col3'}  calRowHeaders={'Row1' 'Row2' 'Row3'}
      settings: SourceProductName=Raptor
  raptor_measurement : S-Function  FunctionName=raptor_sfun_measurement  Parameters=char({dataName,''}), uint8(calDispType), char(enumName), int32(enumValue), double(calGain), double(calOffset), double(calMax), double(calMin), char(calUnit), char(calHelp), char(calFormat), char(calFunction), char(calAccess)  SFunctionDeploymentMode=off  EnableBusSupport=off  mask(Measurement){paramName=[th_nam(1:end-3) 'Tmr'], nameSource=Parameter, calDispType=Number, calEnum={'False', 'True'}, calGain=th_gain, calOffset=0.0, calMax=inf, calMin=-inf, calFormat='0.3', calUnit=th_units, calHelp=['time that gets compared to ' th_nam], calAccess=4, calFunction=th_group, calVisible=on}
      mask prompts: paramName "Name"; nameSource "Name Source"; calDispType "Display as"; calEnum "Enumeration Definition"; calGain "Gain"; calOffset "Offset"; calMax "Max"; calMin "Min"; calFormat "Display Decimal Places"; calUnit "Unit Text"; calHelp "Help Text"; calAccess "Access Level"; calFunction "Function"; calVisible "Visible in Cal"
      mask help: This block is used to display a value in the calibration tool.
      mask init:
      | raptor_sfun_measurement_maskInit;
      settings: MoveFcn=raptor_icon_redraw(gcb);
      mask Help: eval('raptor_help(''raptor_measurement'');')
      mask TypeOptions nameSource: Parameter | Input Wire
      mask Callback nameSource: raptor_sfun_measurement_dlgCb(gcb, 'nameSource');
      mask TypeOptions calDispType: Number | Enumeration | String
      mask Callback calDispType: raptor_sfun_measurement_dlgCb(gcb, 'calDispType');
      mask TypeOptions calAccess: 4 | 3 | 2 | 1
      mask Display: raptor_sfun_measurement_icon;
  RelOp : Outport  VectorParamsAs1DForOutWhenUnconnected=off
  wires:
  Unit Delay2/1 -> Logical Operator2/1
  Rst/1 -> Multiport Switch1/1
  Logical Operator3/1 -> Unit Delay2/1, RelOp/1
  raptor_adjustment/1 -> Relational Operator/2
  Enbl/1 -> Logical Operator1/2
  Logical Operator1/1 -> Multiport Switch/1
  Add/1 -> Multiport Switch/3
  Unit Delay1/1 -> Add/2, Multiport Switch/2
  Constant/1 -> Add/1
  Multiport Switch/1 -> Multiport Switch1/2
  Constant1/1 -> Multiport Switch1/3
  Logical Operator2/1 -> Logical Operator1/1
  Multiport Switch1/1 -> raptor_measurement/1, Unit Delay1/1, Relational Operator/1
  Relational Operator/1 -> Logical Operator3/1
  Logical Operator4/1 -> Logical Operator3/2
  "Rst "/1 -> Logical Operator4/1

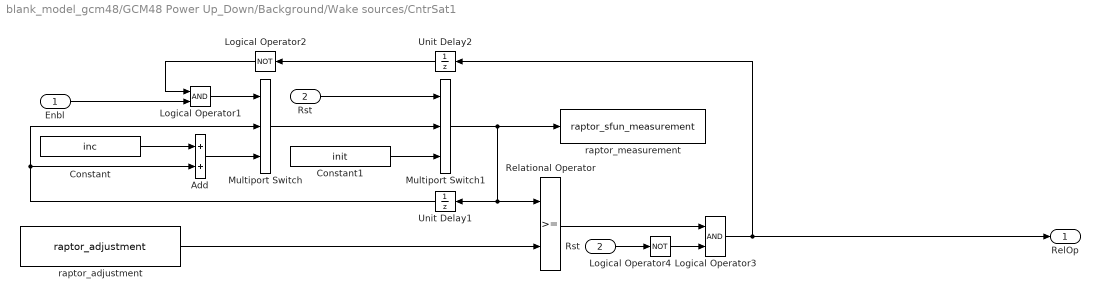
== system blank_model_gcm48/GCM48 Power Up_Down/Background/Wake sources/CntrSat1 ==
  Enbl : Inport
  Rst : Inport  Port=2
  Add : Sum  InputSameDT=on  OutDataTypeStr=Inherit: Same as first input
  Constant : Constant  Value=inc  OutDataTypeStr=uint32
  Constant1 : Constant  Value=init  OutDataTypeStr=uint32
  Logical Operator1 : Logic  OutDataTypeStr=boolean
  Logical Operator2 : Logic  Operator=NOT  Inputs=1  OutDataTypeStr=boolean
  Logical Operator3 : Logic  OutDataTypeStr=boolean
  Logical Operator4 : Logic  Operator=NOT  Inputs=1  OutDataTypeStr=boolean
  Multiport Switch : MultiPortSwitch  DataPortOrder=Zero-based contiguous  Inputs=2  zeroidx=on  InputSameDT=on
  Multiport Switch1 : MultiPortSwitch  DataPortOrder=Zero-based contiguous  Inputs=2  zeroidx=on  InputSameDT=on
  Relational Operator : RelationalOperator  OutDataTypeStr=boolean  RndMeth=Nearest
  "Rst " : InportShadow  Port=2
  Unit Delay1 : UnitDelay  InitialCondition=init  SampleTime=-1  HasFrameUpgradeWarning=on
  Unit Delay2 : UnitDelay  InitialCondition=boolean(0)  SampleTime=-1  HasFrameUpgradeWarning=on
  raptor_adjustment : Raptor_lib/Data Storage/raptor_adjustment  paramName=th_nam  nameSource=Parameter  initValue=5 / th_gain  dataType=uint32  storage=Calibration  calDispType=Number  calEnum={'Disabled', 'Enabled'}  calGain=th_gain  calOffset=0  calMax=inf  calMin=-inf  calFormat='0.3'  calUnit=th_units  calHelp=th_help  calAccess=4  calFunction=th_group  calDispHeaders=off  calColHeaders={'Col1' 'Col2' 'Col3'}  calRowHeaders={'Row1' 'Row2' 'Row3'}
      settings: SourceProductName=Raptor
  raptor_measurement : S-Function  FunctionName=raptor_sfun_measurement  Parameters=char({dataName,''}), uint8(calDispType), char(enumName), int32(enumValue), double(calGain), double(calOffset), double(calMax), double(calMin), char(calUnit), char(calHelp), char(calFormat), char(calFunction), char(calAccess)  SFunctionDeploymentMode=off  EnableBusSupport=off  mask(Measurement){paramName=[th_nam(1:end-3) 'Tmr'], nameSource=Parameter, calDispType=Number, calEnum={'False', 'True'}, calGain=th_gain, calOffset=0.0, calMax=inf, calMin=-inf, calFormat='0.3', calUnit=th_units, calHelp=['time that gets compared to ' th_nam], calAccess=4, calFunction=th_group, calVisible=on}
      mask prompts: paramName "Name"; nameSource "Name Source"; calDispType "Display as"; calEnum "Enumeration Definition"; calGain "Gain"; calOffset "Offset"; calMax "Max"; calMin "Min"; calFormat "Display Decimal Places"; calUnit "Unit Text"; calHelp "Help Text"; calAccess "Access Level"; calFunction "Function"; calVisible "Visible in Cal"
      mask help: This block is used to display a value in the calibration tool.
      mask init:
      | raptor_sfun_measurement_maskInit;
      settings: MoveFcn=raptor_icon_redraw(gcb);
      mask Help: eval('raptor_help(''raptor_measurement'');')
      mask TypeOptions nameSource: Parameter | Input Wire
      mask Callback nameSource: raptor_sfun_measurement_dlgCb(gcb, 'nameSource');
      mask TypeOptions calDispType: Number | Enumeration | String
      mask Callback calDispType: raptor_sfun_measurement_dlgCb(gcb, 'calDispType');
      mask TypeOptions calAccess: 4 | 3 | 2 | 1
      mask Display: raptor_sfun_measurement_icon;
  RelOp : Outport  VectorParamsAs1DForOutWhenUnconnected=off
  wires:
  "Rst "/1 -> Logical Operator4/1
  Logical Operator4/1 -> Logical Operator3/2
  Relational Operator/1 -> Logical Operator3/1
  Multiport Switch1/1 -> Relational Operator/1, Unit Delay1/1, raptor_measurement/1
  Logical Operator2/1 -> Logical Operator1/1
  Constant1/1 -> Multiport Switch1/3
  Multiport Switch/1 -> Multiport Switch1/2
  Constant/1 -> Add/1
  Unit Delay1/1 -> Multiport Switch/2, Add/2
  Add/1 -> Multiport Switch/3
  Logical Operator1/1 -> Multiport Switch/1
  Enbl/1 -> Logical Operator1/2
  raptor_adjustment/1 -> Relational Operator/2
  Logical Operator3/1 -> RelOp/1, Unit Delay2/1
  Rst/1 -> Multiport Switch1/1
  Unit Delay2/1 -> Logical Operator2/1

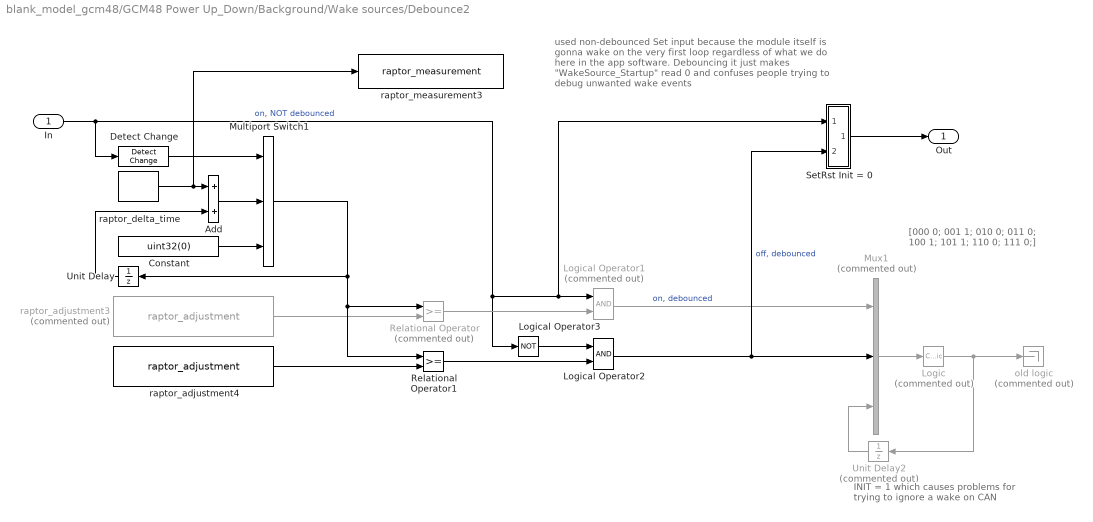
== system blank_model_gcm48/GCM48 Power Up_Down/Background/Wake sources/Debounce2 ==
  note: used non-debounced Set input because the module itself is gonna wake on the very first loop regardless of what we do here in the app software. Debouncing it just makes "WakeSource_Startup" read 0 and confuses people trying to debug unwanted wake events
  note: INIT = 1 which causes problems for trying to ignore a wake on CAN
  note: [000		0;
      |  001		1;
      |  010		0;
      |  011		0;
      |  100		1;
      |  101		1;
      |  110		0;
      |  111		0;]
  In : Inport
  Add : Sum
  Constant : Constant  Value=uint32(0)
  Detect Change : simulink/Logic and Bit Operations/Detect Change  vinit=0  OutDataTypeStr=boolean
  Logic : CombinatorialLogic  Commented=on  TruthTable=[0;1;0;0;1;1;0;0]
  Logical Operator1 : Logic  Commented=on  AllPortsSameDT=off  OutDataTypeStr=boolean
  Logical Operator2 : Logic  AllPortsSameDT=off  OutDataTypeStr=boolean
  Logical Operator3 : Logic  Operator=NOT  Inputs=1  AllPortsSameDT=off  OutDataTypeStr=boolean
  Multiport Switch1 : MultiPortSwitch  DataPortOrder=Zero-based contiguous  Inputs=2  zeroidx=on
  Mux1 : Mux  Commented=on  Inputs=3
  Relational Operator : RelationalOperator  Commented=on  OutDataTypeStr=boolean  RndMeth=Nearest
  Relational Operator1 : RelationalOperator  OutDataTypeStr=boolean  RndMeth=Nearest
  SetRst Init = 0 : Subsystem  mask(SetRst){init=0}
      mask prompts: init "Initial Condition (of output):"
      mask Display:
      | port_label('input', 1, 'S');
      | port_label('input', 2, 'R');
  Unit Delay : UnitDelay  InitialCondition=1  SampleTime=-1  HasFrameUpgradeWarning=on
  Unit Delay2 : UnitDelay  Commented=on  InitialCondition=1  SampleTime=-1  HasFrameUpgradeWarning=on
  old logic : Terminator  Commented=on
  raptor_adjustment3 : Raptor_lib/Data Storage/raptor_adjustment  Commented=on  paramName='KeySwHiTimeThr'  nameSource=Parameter  initValue=200  dataType=uint32  storage=Calibration  calDispType=Number  calEnum={'Active Low', 'Active High'}  calGain=1  calOffset=0  calMax=inf  calMin=-inf  calFormat='-1'  calUnit='milliseconds'  calHelp='State high time threshold'  calAccess=4  calFunction=group  calDispHeaders=off  calColHeaders={'Col1' 'Col2' 'Col3'}  calRowHeaders={'Row1' 'Row2' 'Row3'}
      settings: SourceProductName=Raptor
  raptor_adjustment4 : Raptor_lib/Data Storage/raptor_adjustment  paramName='KeySwLoTimeThr'  nameSource=Parameter  initValue=200  dataType=uint32  storage=Calibration  calDispType=Number  calEnum={'Active Low', 'Active High'}  calGain=1  calOffset=0  calMax=inf  calMin=-inf  calFormat='-1'  calUnit='milliseconds'  calHelp='State low time threshold'  calAccess=4  calFunction=group  calDispHeaders=off  calColHeaders={'Col1' 'Col2' 'Col3'}  calRowHeaders={'Row1' 'Row2' 'Row3'}
      settings: SourceProductName=Raptor
  raptor_delta_time : Raptor_lib/Triggers/raptor_delta_time  unit=milliseconds
      settings: SourceProductName=Raptor
  raptor_measurement3 : Raptor_lib/Data Storage/raptor_measurement  paramName='dt_read'  nameSource=Parameter  calDispType=Number  calEnum={'False', 'True'}  calGain=1.0  calOffset=0.0  calMax=inf  calMin=-inf  calFormat='-1'  calUnit=''  calHelp=''  calAccess=4  calFunction=group  calVisible=on
      settings: SourceProductName=Raptor
  Out : Outport  VectorParamsAs1DForOutWhenUnconnected=off
  wires:
  SetRst Init = 0/1(Bool) -> Out/1
  raptor_adjustment3/1 -> Relational Operator/2
  raptor_adjustment4/1 -> Relational Operator1/2
  raptor_delta_time/1 -> raptor_measurement3/1, Add/1
  Unit Delay/1 -> Add/2
  Logic/1 -> Unit Delay2/1, old logic/1
  Relational Operator1/1 -> Logical Operator2/2
  Constant/1 -> Multiport Switch1/3
  Add/1 -> Multiport Switch1/2
  Multiport Switch1/1 -> Relational Operator1/1, Relational Operator/1, Unit Delay/1
  In/1 -> Logical Operator3/1, Logical Operator1/1, SetRst Init = 0/1(Set), Detect Change/1  "on, NOT debounced"
  Unit Delay2/1 -> Mux1/3
  Mux1/1 -> Logic/1
  Logical Operator1/1 -> Mux1/1  "on, debounced"
  Logical Operator2/1 -> SetRst Init = 0/2(Rst), Mux1/2  "off, debounced"
  Relational Operator/1 -> Logical Operator1/2
  Logical Operator3/1 -> Logical Operator2/1
  Detect Change/1 -> Multiport Switch1/1
